simulink model "regelstrecke_s_function"  (R2023a)
settings: Solver=VariableStepAuto  StartTime=0.0  StopTime=20  RelTol=1e-3
libraries: slident x2
settings Model: Creator=proto  LastModifiedBy=proto
settings DataIOCC: SaveOutput=off  SaveTime=off
settings OptimizationCC: DefaultParameterBehavior=Inlined

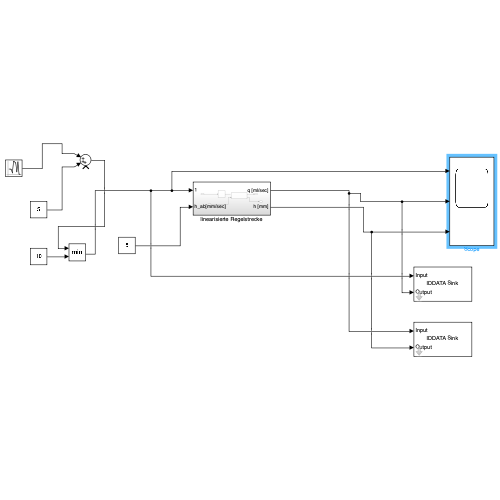
[thumbnail: Simulink's stored preview of the top-level diagram]
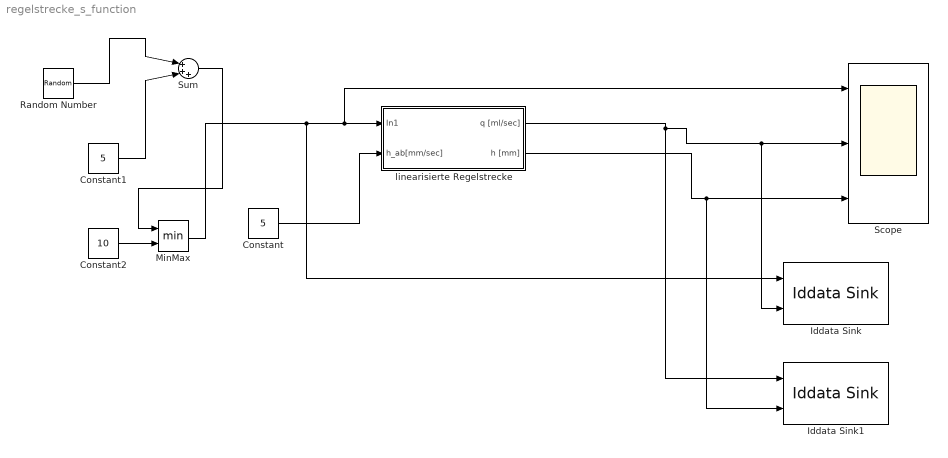
== system regelstrecke_s_function ==
  Constant : Constant  Value=5
  Constant1 : Constant  Value=5
  Constant2 : Constant  Value=10
  Iddata Sink : slident/Iddata Sink  datasetname=V_Q_iddata  Ts=0.1  isu=on  isy=on
  Iddata Sink1 : slident/Iddata Sink  datasetname=q_h_iddata  Ts=0.1  isu=on  isy=on
  MinMax : MinMax  Inputs=2
  Random Number : RandomNumber  Variance=10  SampleTime=0.1
  Scope : Scope  NumInputPorts=3
  Sum : Sum  Inputs=|+++
  linearisierte Regelstrecke : Subsystem
  wires:
  Constant1/1 -> Sum/2
  Random Number/1 -> Sum/1
  linearisierte Regelstrecke/1(q [ml/sec]) -> Iddata Sink1/1, Iddata Sink/2, Scope/2
  linearisierte Regelstrecke/2(h [mm]) -> Iddata Sink1/2, Scope/3
  Constant/1 -> linearisierte Regelstrecke/2(h_ab[mm/sec])
  Constant2/1 -> MinMax/2
  Sum/1 -> MinMax/1
  MinMax/1 -> Iddata Sink/1, Scope/1, linearisierte Regelstrecke/1(In1)

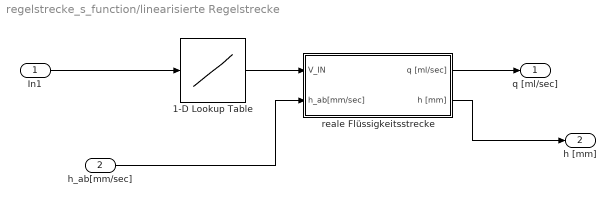
== system regelstrecke_s_function/linearisierte Regelstrecke ==
  In1 : Inport
  h_ab[mm/sec] : Inport  Port=2
  1-D Lookup Table : Lookup_n-D  NumberOfTableDimensions=1  BreakpointsForDimension1=[-11.6,-10.1,-9.0,-7.65,-6.15,-4.4,-2.65,-0.01,0.01,2.65,4.4,6.15,7.65,9.0,10.1,11.6]  Table=[-10,-9,-8,-7,-6,-5,-4,-3,3,4,5,6,7,8,9,10]  InternalRulePriority=Speed  RndMeth=Simplest
  reale Flüssigkeitsstrecke : Subsystem
  q [ml/sec] : Outport
  h [mm] : Outport  Port=2
  wires:
  reale Flüssigkeitsstrecke/2(h [mm]) -> h [mm]/1
  In1/1 -> 1-D Lookup Table/1
  reale Flüssigkeitsstrecke/1(q [ml/sec]) -> q [ml/sec]/1
  h_ab[mm/sec]/1 -> reale Flüssigkeitsstrecke/2(h_ab[mm/sec])
  1-D Lookup Table/1 -> reale Flüssigkeitsstrecke/1(V_IN)

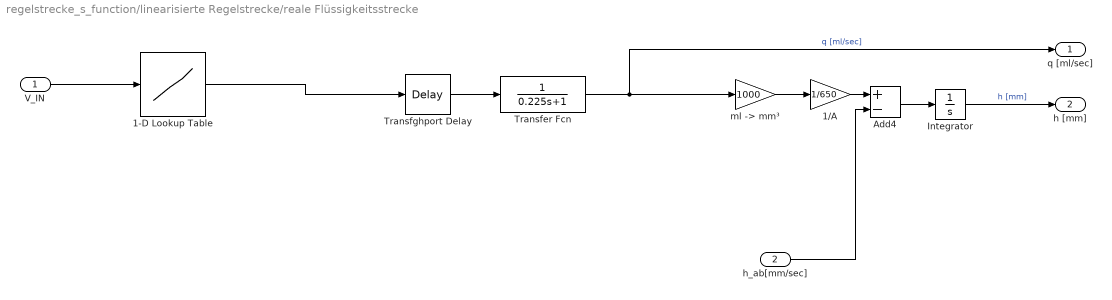
== system regelstrecke_s_function/linearisierte Regelstrecke/reale Flüssigkeitsstrecke ==
  V_IN : Inport
  h_ab[mm/sec] : Inport  Port=2
  1-D Lookup Table : Lookup_n-D  NumberOfTableDimensions=1  BreakpointsForDimension1=[-10,-9,-8,-7,-6,-5,-4,-3,3,4,5,6,7,8,9,10]  Table=[-11.6,-10.1,-9.0,-7.65,-6.15,-4.4,-2.65,0,0,2.65,4.4,6.15,7.65,9.0,10.1,11.6]  InternalRulePriority=Speed  RndMeth=Simplest
  1/A : Gain  Gain=1/650
  Add4 : Sum  Inputs=+-
  Integrator : Integrator  InitialCondition=70  LimitOutput=on  UpperSaturationLimit=153  LowerSaturationLimit=0
  Transfer Fcn : TransferFcn  Denominator=[0.225 1]
  Transfghport Delay : TransportDelay  DelayTime=0.25
  "ml -> mm³" : Gain  Gain=1000
  q [ml/sec] : Outport
  h [mm] : Outport  Port=2
  wires:
  h_ab[mm/sec]/1 -> Add4/2
  V_IN/1 -> 1-D Lookup Table/1
  Integrator/1 -> h [mm]/1  "h [mm]"
  "ml -> mm³"/1 -> 1/A/1
  1-D Lookup Table/1 -> Transfghport Delay/1
  Transfghport Delay/1 -> Transfer Fcn/1
  1/A/1 -> Add4/1
  Transfer Fcn/1 -> q [ml/sec]/1, "ml -> mm³"/1  "q [ml/sec]"
  Add4/1 -> Integrator/1
